simulink model "cw16"  (Simulink 7.0)
settings: Solver=ode4  StartTime=0.0  StopTime=10.0  FixedStep=0.01  RelTol=1e-3
values from neighbouring files (symbols this model uses):
  Beta_rate = 3*(pi/180)    (= 0.0523598775598)    [cw16set.m]
  g = 9.80665    [cw16set.m]
  gainfx = 1    [cw16set.m]
  gainfxtilt = 1    [cw16set.m]
  gainfy = 1    [cw16set.m]
  gainfytilt = 1    [cw16set.m]
  gainfz = 1    [cw16set.m]
  gainp = 1    [cw16set.m]
  gainq = 1    [cw16set.m]
  gainr = 1    [cw16set.m]
  HPomegabphi = 0.0    (= 0)    [cw16set.m]
  HPomegabpsi = 0.0    (= 0)    [cw16set.m]
  HPomegabtheta = 0.0    (= 0)    [cw16set.m]
  HPomegabx = 0.0    (= 0)    [cw16set.m]
  HPomegaby = 0.0    (= 0)    [cw16set.m]
  HPomegabz = 0.2    [cw16set.m]
  HPomeganphi = 1.0    (= 1)    [cw16set.m]
  HPomeganpsi = 1.0    (= 1)    [cw16set.m]
  HPomegantheta = 0.8    [cw16set.m]
  HPomeganx = 0.8    [cw16set.m]
  HPomegany = 1.0    (= 1)    [cw16set.m]
  HPomeganz = 1.0    (= 1)    [cw16set.m]
  HPzetaphi = 1.0    (= 1)    [cw16set.m]
  HPzetapsi = 1.0    (= 1)    [cw16set.m]
  HPzetatheta = 1.0    (= 1)    [cw16set.m]
  HPzetax = 1.0    (= 1)    [cw16set.m]
  HPzetay = 1.0    (= 1)    [cw16set.m]
  HPzetaz = 1.0    (= 1)    [cw16set.m]
  kf = [kfx 0 0; 0 kfy 0; 0 0 kfz]    [cw16set.m]
  Kfeedbackeuler = 0.2    [cw16set.m]
  Kfeedbackeulerrate = 0.5    [cw16set.m]
  Kfeedbackx = 0.5    [cw16set.m]
  Kfeedbackxd = 0.1    [cw16set.m]
  Ktilteuler = 0.2    [cw16set.m]
  Ktilteulerrate = 0.5    [cw16set.m]
  Ktiltrate = 5.0    (= 5)    [cw16set.m]
  kw = [kwp 0 0; 0 kwq 0; 0 0 kwr]    [cw16set.m]
  LPomeganx = 2.0    (= 2)    [cw16set.m]
  LPomegany = 2.0    (= 2)    [cw16set.m]
  LPzetax = 1.0    (= 1)    [cw16set.m]
  LPzetay = 1.0    (= 1)    [cw16set.m]
  LZDERPUGP = 1.2075    [cw16set.m]
  tiltcoordinationmethod = 1    [cw16set.m]
  xref_ac = 0.0    (= 0)    [cw16set.m]
  xref_filt = 0.0    (= 0)    [cw16set.m]
  yref_ac = 0.0    (= 0)    [cw16set.m]
  yref_filt = 0.0    (= 0)    [cw16set.m]
  zref_ac = -1.2075    [cw16set.m]
  zref_filt = 0.0    (= 0)    [cw16set.m]
libraries: simulink x4
(part 2 of 2)

== matlab function Simulator state/calculate position and velocity in filter reference point, for state feedback inside filter ==
  data: x_ugp input double; xd_ugp input double; attsim input double; x_filt output double; refpos input double; xd_filt output double
function [x_filt, xd_filt] = xd_ugp_2_xd_filt(x_ugp, xd_ugp, attsim, refpos)
% This block supports the Embedded MATLAB subset.
% See the help menu for details. 

% This function transforms simulator position and velocities, which are 
% given in the upper gimbal point, to the filter reference position.
% The refpos input is expected to contain:
% [xref_ac; yref_ac; zref_ac; xref_filt; yref_filt; zref_filt]
% All these positions are given relative to the UGP (although in
% this function we're only interested in the difference)

% get some names attached
phi      = attsim(1);
theta    = attsim(2);
psi      = attsim(3);
w        = attsim(4:6);

% gonio stuff
cf = cos(phi); sf = sin(phi); 
ct = cos(theta); st = sin(theta);
cp = cos(psi); sp = sin(psi);

% position to translate over
% filt - ugp(=0)  
dx = refpos(4:6);

% transformation from inertial to body
T = [  cp*ct              sp*ct              -st    ;
      (cp*st*sf - sp*cf) (cp*cf + sp*st*sf) (ct*sf) ;
      (cp*st*cf + sp*sf) (sp*st*cf - cp*sf) (ct*cf) ];

% position from UGP to filter
x_filt = x_ugp + T'*dx;

% velocity from UGP to filter
xd_filt = xd_ugp + T'*cross(w, dx);

== matlab function translate from A/C ref to filter ref in A/C/Embedded MATLAB Function ==
  data: u input double; y output double; refpos input double
function y = fcn(u, refpos)
% This block supports the Embedded MATLAB subset.
% See the help menu for details. 

% This function transforms the filter inputs, which are given in the
% aircraft reference position, to the filter reference position.
% The refpos input is expected to contain:
% [xref_ac; yref_ac; zref_ac; xref_filt; yref_filt; zref_filt]
% All these positions are given relative to the UGP (although in
% this function we're only interested in the difference)

% get some names attached
fx_ac = u(1);
fy_ac = u(2);
fz_ac = u(3);
p     = u(4);
q     = u(5);
r     = u(6);
pd    = u(7);
qd    = u(8);
rd    = u(9);

% position to translate over
% filt-ac
dx = refpos(4) - refpos(1);
dy = refpos(5) - refpos(2);
dz = refpos(6) - refpos(3);

% specific forces
% f_mf = f_ac + wd x r + w x (w x r)
fx_mf = (-r*r - q*q) *dx + (p*q - rd)   *dy + (qd + p*r)   *dz + fx_ac;
fy_mf = (rd + p*q)   *dx + (-r*r - p*p) *dy + (q*r - pd)   *dz + fy_ac;
fz_mf = (p*r - qd)   *dx + (q*r + pd)   *dy + (-q*q - p*p) *dz + fz_ac;

% output
y    = u;
y(1) = fx_mf;
y(2) = fy_mf;
y(3) = fz_mf;

== matlab function translate from filter reference to upper gimbal point (motion base reference)/move inertial acceleration setpoints in MF reference point to UGP reference point ==
  data: xdd_i_mf input double; wd_mf input double; attsim input double; xdd_i_ugp output double; refpos input double
function xdd_i_ugp = xdd_i_mf2xdd_i_ugp(xdd_i_mf, wd_mf, attsim, refpos)
% This block supports the Embedded MATLAB subset.
% See the help menu for details. 

% This function transforms the filter inputs, which are given in the
% aircraft reference position, to the filter reference position.
% The refpos input is expected to contain:
% [xref_ac; yref_ac; zref_ac; xref_filt; yref_filt; zref_filt]
% All these positions are given relative to the UGP (although in
% this function we're only interested in the difference)

% get some names attached
phi      = attsim(1);
theta    = attsim(2);
psi      = attsim(3);
w        = attsim(4:6);

% gonio stuff
cf = cos(phi); sf = sin(phi); 
ct = cos(theta); st = sin(theta);
cp = cos(psi); sp = sin(psi);

% position to translate over
% ugp(=0) - filt
dx = -refpos(4:6);

% transform from inertial to body
% [OS] 20130611 fixed typo (sf->st)
T = [  cp*ct              sp*ct              -st    ;
      (cp*st*sf - sp*cf) (cp*cf + sp*st*sf) (ct*sf) ;
      (cp*st*cf + sp*sf) (sp*st*cf - cp*sf) (ct*cf) ];

xdd_b_mf = T*xdd_i_mf;
  
% translate to UGP
xdd_b_ugp = xdd_b_mf + cross(wd_mf, dx) + cross(w, cross(w, dx));
  
% transform from body to inertial
xdd_i_ugp = T'*xdd_b_ugp;
